simulink model "dq0Invertermeow"  (R2023b)
settings: Solver=VariableStepAuto  StartTime=0.0  StopTime=100  RelTol=1e-3
libraries: eeGeneralControl x7, slpidlib x6, spsAlphaBetaZerotodq0Lib x5, spsCurrentMeasurementLib x5, spsSeriesRLCBranchLib x5, spsIGBTDiodeLib x4, spsabctoAlphaBetaZeroLib x3, spsdq0toAlphaBetaZeroLib x2, spsPLL3phLib x2, simulink x2, spsVoltageMeasurementLib x2, spsACVoltageSourceLib x1
settings Model: Creator=impul  LastModifiedBy=Jia Yee Wong
settings ModelReferenceCC: EnableRefExpFcnMdlSchedulingChecks=on
settings SFSimCC: SimCustomHeaderCode="#include \"referencegen.h\""  SimUserSources=referencegen.c  SimTargetLang=C++

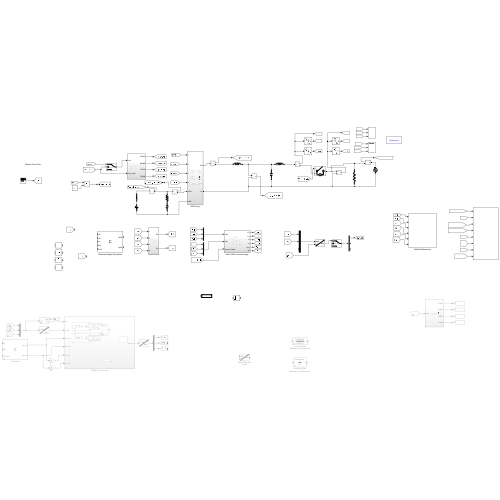
[thumbnail: Simulink's stored preview of the top-level diagram]
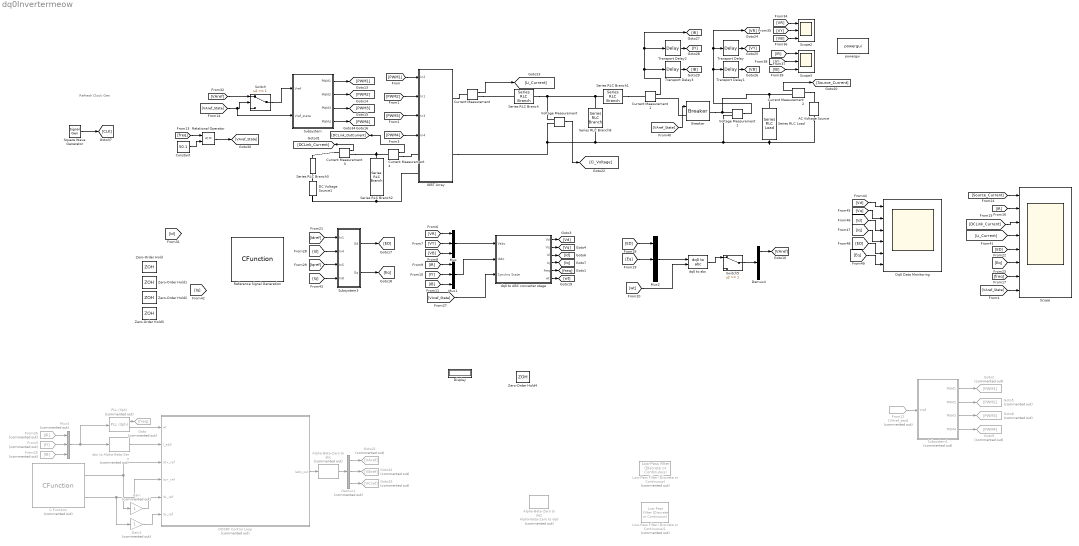
== system dq0Invertermeow ==
  note: Refresh Clock Gen
  AC Voltage Source : spsACVoltageSourceLib/AC Voltage Source  Amplitude=340  Phase=0  Frequency=50  SampleTime=0  Measurements=None  BusType=swing  Pref=0  Qref=0  Qmin=-inf  Qmax=+inf
  Alpha-Beta-Zero to abc : spsAlphaBetaZerotoabcLib/Alpha-Beta-Zero to abc  Commented=on
      settings: LibrarySourceBlock=|
      | sps_lib/Control/Alpha-Beta-Zero
      | to abc
  Alpha-Beta-Zero to dq2 : spsAlphaBetaZerotodq0Lib/Alpha-Beta-Zero to dq0  Commented=on  Alignment=90 degrees behind phase A axis
  Breaker : spsBreakerLib/Breaker  InitialState=0  SwitchingTimes="[1/60  5/60]"  External=on  BreakerResistance=0.00001  SnubberResistance=1e6  SnubberCapacitance=inf  Measurements=None  MoreParameters=on  NoBreakLoop=off
  C Function : CFunction  Commented=on
  Constant : Constant  Value=50.1  SampleTime=0
  Current Measurement{,1..4} (5 alike) : spsCurrentMeasurementLib/Current Measurement  PhasorSimulation=off  OutputType=Complex  PSBequivalent=0
  DC Voltage Source1 : spsDCVoltageSourceLib/DC Voltage Source  Amplitude=400  Measurements=None
  DDSRF Control Loop : Subsystem  Commented=on
  Demux1 : Demux  Commented=on  Outputs=3
  Demux4 : Demux  Outputs=3
  Display : Display
  Dq0 Data Monitoring : Scope  NumInputPorts=6
  From12 : From  Commented=on  GotoTag=VAref_test
  From25 : From  Commented=on  GotoTag=IB
  From26 : From  Commented=on  GotoTag=IR
  From5 : From  Commented=on  GotoTag=IY
  Gain : Gain  Commented=on
  Gain1 : Gain  Commented=on
  Goto : Goto  Commented=on  GotoTag=freq
  Goto2 : Goto  Commented=on  GotoTag=PWM1
  Goto21 : Goto  Commented=on  GotoTag=VAref
  Goto32 : Goto  Commented=on  GotoTag=VBref
  Goto33 : Goto  Commented=on  GotoTag=VCref
  Goto5 : Goto  Commented=on  GotoTag=PWM2
  Goto8 : Goto  Commented=on  GotoTag=PWM3
  Goto9 : Goto  Commented=on  GotoTag=PWM4
  IGBT Array : Subsystem
  Low-Pass Filter (Discrete or Continuous) : eeGeneralControl/Low-Pass Filter (Discrete or Continuous)  Commented=on  K=1  T=2*pi*1  B=inf  A=-inf  init_option=Inherited from block input  x0=0  Ts=0
  Low-Pass Filter (Discrete or Continuous)1 : eeGeneralControl/Low-Pass Filter (Discrete or Continuous)  Commented=on  K=1  T=1  B=inf  A=-inf  init_option=Inherited from block input  x0=0  Ts=0
  Mux : Mux  Inputs=3
  Mux1 : Mux  Inputs=3
  Mux2 : Mux  Inputs=3
  Mux3 : Mux  Commented=on  Inputs=3
  PLL (3ph) : spsPLL3phLib/PLL (3ph)  Commented=on  Fmin=45  Par_Init=[0, 60]  ParK=[180, 3200, 1]  TcD=1e-4  MaxRateChangeFreq=12  FilterCutOffFreq=25  Ts=0  AGC=on
  Reference Signal Generation : CFunction
  Relational Operator : RelationalOperator  Operator=<=  OutDataTypeStr=boolean  RndMeth=Simplest  InputSameDT=off
  Scope : Scope  NumInputPorts=8
  Scope2 : Scope  NumInputPorts=3
  Scope3 : Scope  NumInputPorts=3
  Series RLC Branch : spsSeriesRLCBranchLib/Series RLC Branch  LConnTagsString=__new0  RConnTagsString=__new0  BranchType=L  Resistance=1  Inductance=20.4e-3  SetiL0=off  InitialCurrent=0  Capacitance=1e-6  Setx0=off  InitialVoltage=0  Measurements=None
  Series RLC Branch1 : spsSeriesRLCBranchLib/Series RLC Branch  LConnTagsString=__new0  RConnTagsString=__new0  BranchType=L  Resistance=1  Inductance=148.336e-6  SetiL0=off  InitialCurrent=0  Capacitance=1e-6  Setx0=off  InitialVoltage=0  Measurements=None
  Series RLC Branch2 : spsSeriesRLCBranchLib/Series RLC Branch  LConnTagsString=__new0  RConnTagsString=__new0  BranchType=RC  Resistance=0.1  Inductance=0  SetiL0=off  InitialCurrent=0  Capacitance=1e-6  Setx0=off  InitialVoltage=0  Measurements=None
  Series RLC Branch3 : spsSeriesRLCBranchLib/Series RLC Branch  LConnTagsString=__new0  RConnTagsString=__new0  BranchType=R  Resistance=50  Inductance=0  SetiL0=off  InitialCurrent=0  Capacitance=1e-6  Setx0=off  InitialVoltage=0  Measurements=None
  Series RLC Branch8 : spsSeriesRLCBranchLib/Series RLC Branch  LConnTagsString=__new0  RConnTagsString=__new0  BranchType=C  Resistance=1  Inductance=100e-6  SetiL0=off  InitialCurrent=0  Capacitance=5.526e-6  Setx0=off  InitialVoltage=0  Measurements=None
  Series RLC Load : spsSeriesRLCLoadLib/Series RLC Load  LConnTagsString=a  RConnTagsString=__new0  NominalVoltage=240  NominalFrequency=50  ActivePower=2e3  InductivePower=0  CapacitivePower=0  Setx0=off  InitialVoltage=240  SetiL0=off  InitialCurrent=10  Measurements=None  LoadType=constant PQ
  Square Wave Generator : SignalGenerator  WaveForm=square  Frequency=10e3
  Subsystem : Subsystem
  Subsystem1 : Subsystem  Commented=on
  Subsystem3 : Subsystem
  Switch : Switch  Threshold=1  SaturateOnIntegerOverflow=off  InputSameDT=off
  Switch5 : Switch  Threshold=1  SaturateOnIntegerOverflow=off  InputSameDT=off
  Transport Delay : TransportDelay  DelayTime=6.67e-3  BufferSize=4096
  Transport Delay1 : TransportDelay  DelayTime=13.34e-3  BufferSize=5120
  Transport Delay2 : TransportDelay  DelayTime=6.67e-3  BufferSize=4096
  Transport Delay3 : TransportDelay  DelayTime=13.34e-3  BufferSize=4096
  Voltage Measurement : spsVoltageMeasurementLib/Voltage Measurement  PhasorSimulation=off  OutputType=Complex  PSBequivalent=0
  Voltage Measurement1 : spsVoltageMeasurementLib/Voltage Measurement  PhasorSimulation=off  OutputType=Complex  PSBequivalent=0
  Zero-Order Hold{,1..3} (4 alike) : ZeroOrderHold  SampleTime=-1
  Zero-Order Hold4 : ZeroOrderHold  SampleTime=10e-3
  abc to Alpha-Beta-Zero : spsabctoAlphaBetaZeroLib/abc to Alpha-Beta-Zero  Commented=on
  dq0 to ABC converter stage : Subsystem
  dq0 to abc : spsdq0toabcLib/dq0 to abc  Alignment=90 degrees behind phase A axis
  powergui : spspowerguiLib/powergui  Priority=1  SimulationMode=Continuous  SampleTime=50e-6  frequency=60  Iterations=50  frequencyindice=0  Pbase=100e6  ErrMax=1e-4  UnitsV=kV  UnitsW=MW  buscounter=0  FunctionMessages=off  echomessages=off  EnableUseOfTLC=off  CurrentSourceSwitches=off  DisableSnubberDevices=off  DisableRonSwitches=off  DisableVfSwitches=off  DisplayEquations=off  AutomaticDiscreteSolvers=off  SolverType=Tustin/Backward Euler (TBE)  Interpol=off  ExternalGateDelay=off  methode=off  Ts=100  x0status=blocks  SPID=on  SwTol=0  HookPort=off  NonlinearTolerance=1e-4  nMaxIteration=100  ContinueOnMaxIteration=off  RestoreLinks=warning  ResistiveCurrentMeasurement=off  Frange=[0:2:500]  Ylog=off  Xlog=on  ShowGrid=off  save=off  variable=ZData  structure=0  ZoomFFT=off  StartTime=0.0  cycles=1  DisplayStyle=1  fundamental=60  FreqAxis=off  MaxFrequency=1000  frequencyindicesteady=1  RmsSteady=1  display=off
  wires:
  [PWM1] -> IGBT Array/1(In2)
  [PWM2] -> IGBT Array/2(In1)
  [PWM3] -> IGBT Array/3(In3)
  [PWM4] -> IGBT Array/4(In4)
  [ED] -> Mux2/1
  [Eq] -> Mux2/2
  [wt] -> dq0 to abc/2
  Mux2/1 -> dq0 to abc/1
  Demux4/1 -> [VAref]
  Voltage Measurement/1 -> [Ci_Voltage]
  Transport Delay1/1 -> [VB]
  Transport Delay/1 -> [VY]
  Subsystem/1(PWM1) -> [PWM1]
  Subsystem/2(PWM2) -> [PWM2]
  Subsystem/3(PWM3) -> [PWM3]
  Subsystem/4(PWM4) -> [PWM4]
  Transport Delay2/1 -> [IY]
  Transport Delay3/1 -> [IB]
  Current Measurement/1 -> [Li_Current]
  Current Measurement1/1 -> [IR], Transport Delay2/1, Transport Delay3/1
  Current Measurement2/1 -> [Source_Current]
  Subsystem1/2(PWM2) -> Goto5/1
  From12/1 -> Subsystem1/1(Vref)
  Subsystem1/4(PWM4) -> Goto9/1
  Subsystem1/3(PWM3) -> Goto8/1
  Subsystem1/1(PWM1) -> Goto2/1
  Voltage Measurement1/1 -> [VR], Transport Delay/1, Transport Delay1/1
  [VAref] -> Switch/1
  [freq] -> Relational Operator/1
  Constant/1 -> Relational Operator/2
  Current Measurement3/1 -> [DCLink_Current]
  [Eq] -> Scope/6
  [ED] -> Scope/5
  [VAref_State] -> Scope/8
  Switch/1 -> Subsystem/1(Vref)
  [VAref_State] -> Subsystem/2(Vref_state), Switch/2
  [Source_Current] -> Scope/1
  Switch5/1 -> Demux4/1
  dq0 to abc/1 -> Switch5/1
  [VR] -> Scope2/1
  [VY] -> Scope2/2
  [VB] -> Scope2/3
  [IR] -> Scope3/1
  [IY] -> Scope3/2
  [IB] -> Scope3/3
  [Vd] -> Dq0 Data Monitoring/1
  [Vq] -> Dq0 Data Monitoring/2
  [Id] -> Dq0 Data Monitoring/3
  [Iq] -> Dq0 Data Monitoring/4
  [ED] -> Dq0 Data Monitoring/5
  [Eq] -> Dq0 Data Monitoring/6
  [VAref_State] -> Breaker/1
  [freq] -> Scope/7
  [Li_Current] -> Scope/4
  [IR] -> Scope/2
  [DCLink_Current] -> Scope/3
  Relational Operator/1 -> [VAref_State]
  Subsystem3/1(Ed) -> [ED]
  Subsystem3/2(Eq) -> [Eq]
  [VR] -> Mux/1
  [VB] -> Mux/3
  [IB] -> Mux1/3
  Mux1/1 -> dq0 to ABC converter stage/2(IAbc)
  [IY] -> Mux1/2
  Mux/1 -> dq0 to ABC converter stage/1(Vabc)
  [IR] -> Mux1/1
  [VY] -> Mux/2
  dq0 to ABC converter stage/2(Vq) -> [Vq]
  dq0 to ABC converter stage/1(Vd) -> [Vd]
  dq0 to ABC converter stage/3(Id) -> [Id]
  dq0 to ABC converter stage/4(Iq) -> [Iq]
  dq0 to ABC converter stage/6(wt) -> [wt]
  dq0 to ABC converter stage/5(freq) -> [freq]
  DDSRF Control Loop/1(Iabc_out) -> Alpha-Beta-Zero to abc/1
  PLL (3ph)/2 -> DDSRF Control Loop/1(wt)
  PLL (3ph)/1 -> Goto/1
  abc to Alpha-Beta-Zero/1 -> DDSRF Control Loop/2(I_ab0)
  From25/1 -> Mux3/3
  Mux3/1 -> PLL (3ph)/1, abc to Alpha-Beta-Zero/1
  From5/1 -> Mux3/2
  From26/1 -> Mux3/1
  C Function/2 -> Gain1/1, DDSRF Control Loop/4(Iq+_ref)
  Gain/1 -> DDSRF Control Loop/5(Id-_ref)
  C Function/1 -> Gain/1, DDSRF Control Loop/3(Id+_ref)
  Gain1/1 -> DDSRF Control Loop/6(Iq-_ref)
  Demux1/3 -> Goto33/1
  Demux1/2 -> Goto32/1
  Demux1/1 -> Goto21/1
  Alpha-Beta-Zero to abc/1 -> Demux1/1
  [VAref_State] -> dq0 to ABC converter stage/3(Synchro State)
  Current Measurement4/1 -> [DCLink_OutCurrent]
  [Idref] -> Subsystem3/1(In1)
  [Id] -> Subsystem3/2(In4)
  [Iqref] -> Subsystem3/3(In5)
  [Iq] -> Subsystem3/4(In8)
  Square Wave Generator/1 -> [CLK]
  connections:
  Series RLC Branch/RConn1 -- Voltage Measurement/LConn1 -- Series RLC Branch8/LConn1 -- Series RLC Branch1/LConn1
  Series RLC Branch2/RConn1 -- DC Voltage Source1/LConn1 -- IGBT Array/LConn2
  IGBT Array/RConn2 -- Voltage Measurement/LConn2 -- AC Voltage Source/LConn1 -- Series RLC Load/RConn1 -- Voltage Measurement1/LConn2 -- Series RLC Branch8/RConn1
  IGBT Array/RConn1 -- Current Measurement/LConn1
  Current Measurement/RConn1 -- Series RLC Branch/LConn1
  Series RLC Branch1/RConn1 -- Current Measurement1/LConn1
  Current Measurement2/LConn1 -- AC Voltage Source/RConn1
  Current Measurement2/RConn1 -- Breaker/RConn1 -- Voltage Measurement1/LConn1 -- Series RLC Load/LConn1
  Current Measurement3/RConn1 -- Series RLC Branch2/LConn1 -- Current Measurement4/LConn1
  Series RLC Branch3/RConn1 -- DC Voltage Source1/RConn1
  Breaker/LConn1 -- Current Measurement1/RConn1
  Current Measurement3/LConn1 -- Series RLC Branch3/LConn1
  Current Measurement4/RConn1 -- IGBT Array/LConn1

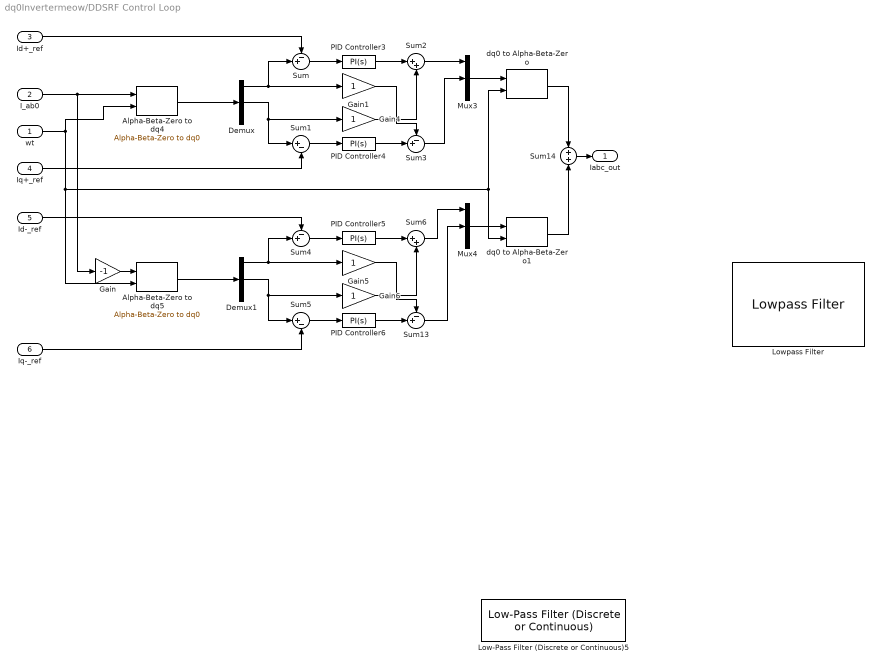
== system dq0Invertermeow/DDSRF Control Loop ==
  wt : Inport
  I_ab0 : Inport  Port=2
  Id+_ref : Inport  Port=3
  Iq+_ref : Inport  Port=4
  Id-_ref : Inport  Port=5
  Iq-_ref : Inport  Port=6
  Alpha-Beta-Zero to dq4 : spsAlphaBetaZerotodq0Lib/Alpha-Beta-Zero to dq0  Alignment=90 degrees behind phase A axis
  Alpha-Beta-Zero to dq5 : spsAlphaBetaZerotodq0Lib/Alpha-Beta-Zero to dq0  Alignment=90 degrees behind phase A axis
  Demux : Demux  Outputs=3
  Demux1 : Demux  Outputs=3
  Gain : Gain  Gain=-1
  Gain{1,4..6} (4 alike) : Gain
  Low-Pass Filter (Discrete or Continuous)5 : eeGeneralControl/Low-Pass Filter (Discrete or Continuous)  K=1  T=2*pi*50  B=inf  A=-inf  init_option=Inherited from block input  x0=0  Ts=0
  Lowpass Filter : dspfdesign/Lowpass Filter  FilterType=FIR  DesignForMinimumOrder=on  FilterOrder=50  PassbandFrequency=8e3  StopbandFrequency=12e3  PassbandRipple=0.1  StopbandAttenuation=80  SampleRateMode=Specify on dialog  SampleRate=44100  SimulateUsing=Interpreted execution  roundingMode=Floor  coeffsDataTypeStr=fixdt(1,16)
  Mux3 : Mux  Inputs=3
  Mux4 : Mux  Inputs=3
  PID Controller{3..6} (4 alike) : slpidlib/PID Controller  Controller=PI  Form=Parallel  TimeDomain=Continuous-time  UseExternalTs=off  SampleTime=-1  IntegratorMethod=Forward Euler  FilterMethod=Forward Euler  ControllerParametersSource=internal  P=1  I=1  UseKiTs=off  D=0  N=100  UseFilter=on  TunerSelectOption=Transfer Function Based (PID Tuner App)  InitialConditionSource=internal  InitialConditionForIntegrator=0  InitialConditionForFilter=0  DifferentiatorICPrevScaledInput=0  ExternalReset=none  TrackingMode=off  Kt=1  LimitOutput=off  SatLimitsSource=internal  UpperSaturationLimit=inf  LowerSaturationLimit=-inf  LinearizeAsGain=on  AntiWindupMode=none  Kb=1  LimitIntegrator=off  UpperIntegratorSaturationLimit=inf  LowerIntegratorSaturationLimit=-inf  POutMin=[]  POutMax=[]  IOutMin=[]  IOutMax=[]  DOutMin=[]  DOutMax=[]  NOutMin=[]  NOutMax=[]  SumOutMin=[]  SumOutMax=[]  SaturationOutMin=[]  SaturationOutMax=[]  PParamMin=[]  PParamMax=[]  IParamMin=[]  IParamMax=[]  DParamMin=[]  DParamMax=[]  NParamMin=[]  NParamMax=[]  KbParamMin=[]  KbParamMax=[]  KtParamMin=[]  KtParamMax=[]  KbOutMin=[]  KbOutMax=[]  KtOutMin=[]  KtOutMax=[]  IntegratorOutMin=[]  IntegratorOutMax=[]  FilterOutMin=[]  FilterOutMax=[]  SumI1OutMin=[]  SumI1OutMax=[]  SumI2OutMin=[]  SumI2OutMax=[]  SumI3OutMin=[]  SumI3OutMax=[]  SumI4OutMin=[]  SumI4OutMax=[]  SumDOutMin=[]  SumDOutMax=[]  DifferentiatorOutMin=[]  DifferentiatorOutMax=[]  FilterDiffOutCoefMin=[]  FilterDiffOutCoefMax=[]  ReciprocalOutMin=[]  ReciprocalOutMax=[]  SumDenOutMin=[]  SumDenOutMax=[]  SumNumOutMin=[]  SumNumOutMax=[]  DivideOutMin=[]  DivideOutMax=[]  UdiffTsProdOutMin=[]  UdiffTsProdOutMax=[]  NTsProdOutMin=[]  NTsProdOutMax=[]  UintegralTsProdOutMin=[]  UintegralTsProdOutMax=[]  UngainTsProdOutMin=[]  UngainTsProdOutMax=[]  ClampingZeroOutDataTypeStr=Inherit: Inherit via back propagation  ClampingZeroOutMin=[]  ClampingZeroOutMax=[]  FilterDenConstantOutDataTypeStr=Inherit: Inherit via back propagation  FilterDenConstantOutMin=[]  FilterDenConstantOutMax=[]  PCopyOutDataTypeStr=Inherit: Inherit via back propagation  PCopyOutMin=[]  PCopyOutMax=[]  NCopyOutDataTypeStr=Inherit: Inherit via back propagation  NCopyOutMin=[]  NCopyOutMax=[]  IntegratorContinuousStateAttributes=''  IntegratorStateMustResolveToSignalObject=off  IntegratorRTWStateStorageClass=Auto  FilterContinuousStateAttributes=''  FilterStateMustResolveToSignalObject=off  FilterRTWStateStorageClass=Auto  ParallelPVariant=InternalParameters  IdealPVariant=Disabled  IVariant=InternalParameters  DVariant=Disabled  IntegratorVariant=Continuous  SatVariant=Disabled  AWVariant=Passthrough  PCopyVariant=Disabled  TRVariant=Disabled  FdbkBlocksVariant=Forward  IdealPFdbkVariant=Disabled  SatFdbkVariant=Disabled  DerivativeFilterVariant=Disabled  NVariant=Disabled  NCopyVariant=Disabled_SignalSpec  FilterICVariant=Disabled  IntegratorICVariant=InternalICs  ExternalResetVariant=Disabled  TRSumVariant=Passthrough  SumFdbkVariant=Disabled  SumVariant=Sum_PI  TsampFilterVariant=InternalTs  TsampNgainVariant=Passthrough  TsampIntegralVariant=Disabled_SignalSpec  ExternalSaturationOutDataTypeStr=Inherit: Same as second input
  Sum{,3..4,13} (4 alike) : Sum  Inputs=-+|
  Sum1 : Sum  Inputs=|+-
  Sum14 : Sum  Inputs=+|+
  Sum2 : Sum  Inputs=|++
  Sum5 : Sum  Inputs=|+-
  Sum6 : Sum  Inputs=|++
  dq0 to Alpha-Beta-Zero : spsdq0toAlphaBetaZeroLib/dq0 to Alpha-Beta-Zero  Alignment=90 degrees behind phase A axis
  dq0 to Alpha-Beta-Zero1 : spsdq0toAlphaBetaZeroLib/dq0 to Alpha-Beta-Zero  Alignment=90 degrees behind phase A axis
  Iabc_out : Outport
  wires:
  Gain/1 -> Alpha-Beta-Zero to dq5/1
  Gain5/1 -> Sum13/1
  Mux3/1 -> dq0 to Alpha-Beta-Zero/1
  PID Controller3/1 -> Sum2/1
  Id-_ref/1 -> Sum4/1
  Demux1/1 -> Gain5/1, Sum4/2
  Demux/1 -> Gain1/1, Sum/2
  Demux/2 -> Gain4/1, Sum1/1
  Sum4/1 -> PID Controller5/1
  dq0 to Alpha-Beta-Zero/1 -> Sum14/1
  PID Controller6/1 -> Sum13/2
  Demux1/2 -> Gain6/1, Sum5/1
  Alpha-Beta-Zero to dq4/1 -> Demux/1
  PID Controller4/1 -> Sum3/2
  Mux4/1 -> dq0 to Alpha-Beta-Zero1/1
  Id+_ref/1 -> Sum/1
  Gain1/1 -> Sum3/1
  Sum/1 -> PID Controller3/1
  Sum1/1 -> PID Controller4/1
  Sum6/1 -> Mux4/1
  Sum2/1 -> Mux3/1
  Iq-_ref/1 -> Sum5/2
  I_ab0/1 -> Alpha-Beta-Zero to dq4/1, Gain/1
  Iq+_ref/1 -> Sum1/2
  Sum3/1 -> Mux3/2
  wt/1 -> Alpha-Beta-Zero to dq4/2, dq0 to Alpha-Beta-Zero/2, dq0 to Alpha-Beta-Zero1/2, Alpha-Beta-Zero to dq5/2
  Alpha-Beta-Zero to dq5/1 -> Demux1/1
  Sum5/1 -> PID Controller6/1
  dq0 to Alpha-Beta-Zero1/1 -> Sum14/2
  Gain6/1 -> Sum6/2
  Sum13/1 -> Mux4/2
  Gain4/1 -> Sum2/2
  PID Controller5/1 -> Sum6/1
  Sum14/1 -> Iabc_out/1

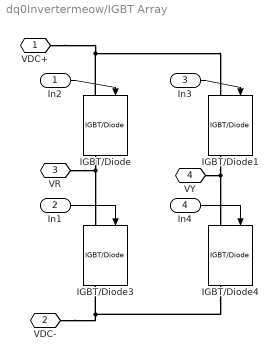
== system dq0Invertermeow/IGBT Array ==
  In2 : Inport
  In1 : Inport  Port=2
  In3 : Inport  Port=3
  In4 : Inport  Port=4
  IGBT/Diode{,1,3..4} (4 alike) : spsIGBTDiodeLib/IGBT//Diode  Ron=1e-3  Rs=1e5  Cs=inf  Measurements=on
  VDC+ : PMIOPort  Side=Left
  VDC- : PMIOPort  Port=2  Side=Left
  VR : PMIOPort  Port=3  Side=Right
  VY : PMIOPort  Port=4  Side=Right
  wires:
  In1/1 -> IGBT/Diode3/1
  In4/1 -> IGBT/Diode4/1
  In3/1 -> IGBT/Diode1/1
  In2/1 -> IGBT/Diode/1
  connections:
  IGBT/Diode4/RConn1 -- VDC-/RConn1 -- IGBT/Diode3/RConn1
  IGBT/Diode/RConn1 -- VR/RConn1 -- IGBT/Diode3/LConn1
  IGBT/Diode1/RConn1 -- VY/RConn1 -- IGBT/Diode4/LConn1
  IGBT/Diode/LConn1 -- VDC+/RConn1 -- IGBT/Diode1/LConn1

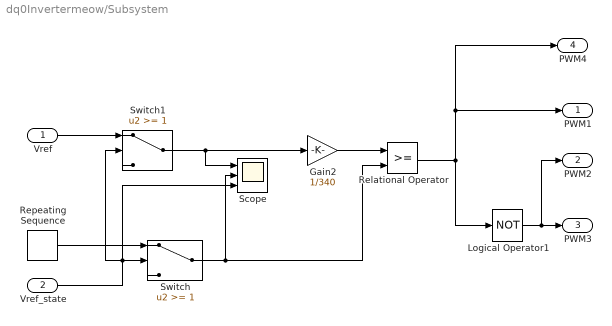
== system dq0Invertermeow/Subsystem ==
  Vref : Inport
  Vref_state : Inport  Port=2
  Gain2 : Gain  Gain=1/340
  Logical Operator1 : Logic  Operator=NOT  AllPortsSameDT=off  OutDataTypeStr=boolean
  Relational Operator : RelationalOperator  OutDataTypeStr=boolean  RndMeth=Simplest  InputSameDT=off
  Repeating Sequence : simulink/Sources/Repeating Sequence  rep_seq_t=[0 0.00005 0.0001]  rep_seq_y=[-1 1 -1]
  Scope : Scope  NumInputPorts=3
  Switch : Switch  Threshold=1  SaturateOnIntegerOverflow=off  InputSameDT=off
  Switch1 : Switch  Threshold=1  SaturateOnIntegerOverflow=off  InputSameDT=off
  PWM1 : Outport
  PWM2 : Outport  Port=2
  PWM3 : Outport  Port=3
  PWM4 : Outport  Port=4
  wires:
  Gain2/1 -> Relational Operator/1
  Relational Operator/1 -> Logical Operator1/1, PWM1/1, PWM4/1
  Logical Operator1/1 -> PWM2/1, PWM3/1
  Repeating Sequence/1 -> Switch/1
  Switch/1 -> Scope/2, Relational Operator/2
  Vref_state/1 -> Scope/3, Switch1/2, Switch/2
  Switch1/1 -> Gain2/1, Scope/1
  Vref/1 -> Switch1/1

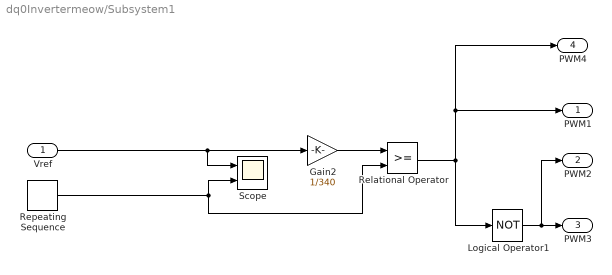
== system dq0Invertermeow/Subsystem1 ==
  Vref : Inport
  Gain2 : Gain  Gain=1/340
  Logical Operator1 : Logic  Operator=NOT  AllPortsSameDT=off  OutDataTypeStr=boolean
  Relational Operator : RelationalOperator  OutDataTypeStr=boolean  RndMeth=Simplest  InputSameDT=off
  Repeating Sequence : simulink/Sources/Repeating Sequence  rep_seq_t=[0 0.00005 0.0001]  rep_seq_y=[-1 1 -1]
  Scope : Scope  NumInputPorts=2
  PWM1 : Outport
  PWM2 : Outport  Port=2
  PWM3 : Outport  Port=3
  PWM4 : Outport  Port=4
  wires:
  Repeating Sequence/1 -> Scope/2, Relational Operator/2
  Gain2/1 -> Relational Operator/1
  Relational Operator/1 -> Logical Operator1/1, PWM1/1, PWM4/1
  Logical Operator1/1 -> PWM2/1, PWM3/1
  Vref/1 -> Scope/1, Gain2/1

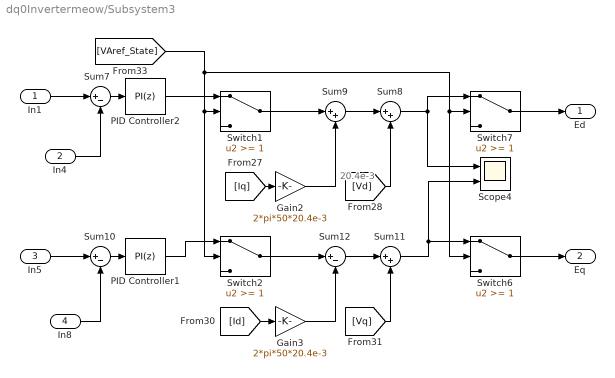
== system dq0Invertermeow/Subsystem3 ==
  note: 20.4e-3
  In1 : Inport
  In4 : Inport  Port=2
  In5 : Inport  Port=3
  In8 : Inport  Port=4
  Gain2 : Gain  Gain=2*pi*50*20.4e-3
  Gain3 : Gain  Gain=2*pi*50*20.4e-3
  PID Controller1 : slpidlib/PID Controller  Controller=PI  Form=Ideal  TimeDomain=Discrete-time  UseExternalTs=off  SampleTime=1e-4  IntegratorMethod=Forward Euler  FilterMethod=Forward Euler  ControllerParametersSource=internal  P=10  I=0.07  UseKiTs=on  D=0.2  N=100  UseFilter=on  TunerSelectOption=Transfer Function Based (PID Tuner App)  InitialConditionSource=internal  InitialConditionForIntegrator=0  InitialConditionForFilter=0  DifferentiatorICPrevScaledInput=0  ExternalReset=none  TrackingMode=off  Kt=1  LimitOutput=on  SatLimitsSource=internal  UpperSaturationLimit=200  LowerSaturationLimit=-200  LinearizeAsGain=on  AntiWindupMode=clamping  Kb=1  LimitIntegrator=off  UpperIntegratorSaturationLimit=inf  LowerIntegratorSaturationLimit=-inf  POutMin=[]  POutMax=[]  IOutMin=[]  IOutMax=[]  DOutMin=[]  DOutMax=[]  NOutMin=[]  NOutMax=[]  SumOutMin=[]  SumOutMax=[]  SaturationOutMin=[]  SaturationOutMax=[]  PParamMin=[]  PParamMax=[]  IParamMin=[]  IParamMax=[]  DParamMin=[]  DParamMax=[]  NParamMin=[]  NParamMax=[]  KbParamMin=[]  KbParamMax=[]  KtParamMin=[]  KtParamMax=[]  KbOutMin=[]  KbOutMax=[]  KtOutMin=[]  KtOutMax=[]  IntegratorOutMin=[]  IntegratorOutMax=[]  FilterOutMin=[]  FilterOutMax=[]  SumI1OutMin=[]  SumI1OutMax=[]  SumI2OutMin=[]  SumI2OutMax=[]  SumI3OutMin=[]  SumI3OutMax=[]  SumI4OutMin=[]  SumI4OutMax=[]  SumDOutMin=[]  SumDOutMax=[]  DifferentiatorOutMin=[]  DifferentiatorOutMax=[]  FilterDiffOutCoefMin=[]  FilterDiffOutCoefMax=[]  ReciprocalOutMin=[]  ReciprocalOutMax=[]  SumDenOutMin=[]  SumDenOutMax=[]  SumNumOutMin=[]  SumNumOutMax=[]  DivideOutMin=[]  DivideOutMax=[]  UdiffTsProdOutMin=[]  UdiffTsProdOutMax=[]  NTsProdOutMin=[]  NTsProdOutMax=[]  UintegralTsProdOutMin=[]  UintegralTsProdOutMax=[]  UngainTsProdOutMin=[]  UngainTsProdOutMax=[]  ClampingZeroOutDataTypeStr=Inherit: Inherit via back propagation  ClampingZeroOutMin=[]  ClampingZeroOutMax=[]  FilterDenConstantOutDataTypeStr=Inherit: Inherit via back propagation  FilterDenConstantOutMin=[]  FilterDenConstantOutMax=[]  PCopyOutDataTypeStr=Inherit: Inherit via back propagation  PCopyOutMin=[]  PCopyOutMax=[]  NCopyOutDataTypeStr=Inherit: Inherit via back propagation  NCopyOutMin=[]  NCopyOutMax=[]  IntegratorContinuousStateAttributes=''  IntegratorStateMustResolveToSignalObject=off  IntegratorRTWStateStorageClass=Auto  FilterContinuousStateAttributes=''  FilterStateMustResolveToSignalObject=off  FilterRTWStateStorageClass=Auto  ParallelPVariant=Passthrough  IdealPVariant=InternalParameters  IVariant=InternalParameters  DVariant=Disabled  IntegratorVariant=Discrete  SatVariant=Enabled  AWVariant=DiscClampingIdeal  PCopyVariant=InternalParamsIdeal  TRVariant=Disabled  FdbkBlocksVariant=Forward  IdealPFdbkVariant=Disabled  SatFdbkVariant=Disabled  DerivativeFilterVariant=Disabled  NVariant=Disabled  NCopyVariant=Disabled_SignalSpec  FilterICVariant=Disabled  IntegratorICVariant=InternalICs  ExternalResetVariant=Disabled  TRSumVariant=Passthrough  SumFdbkVariant=Disabled  SumVariant=Sum_PI  TsampFilterVariant=InternalTs  TsampNgainVariant=Passthrough  TsampIntegralVariant=Disabled_SignalSpec  ExternalSaturationOutDataTypeStr=Inherit: Same as second input
  PID Controller2 : slpidlib/PID Controller  Controller=PI  Form=Parallel  TimeDomain=Discrete-time  UseExternalTs=off  SampleTime=1e-4  IntegratorMethod=Forward Euler  FilterMethod=Forward Euler  ControllerParametersSource=internal  P=10  I=0.07  UseKiTs=on  D=0.2  N=100  UseFilter=on  TunerSelectOption=Transfer Function Based (PID Tuner App)  InitialConditionSource=internal  InitialConditionForIntegrator=0  InitialConditionForFilter=0  DifferentiatorICPrevScaledInput=0  ExternalReset=none  TrackingMode=off  Kt=1  LimitOutput=on  SatLimitsSource=internal  UpperSaturationLimit=200  LowerSaturationLimit=-200  LinearizeAsGain=on  AntiWindupMode=back-calculation  Kb=1  LimitIntegrator=off  UpperIntegratorSaturationLimit=inf  LowerIntegratorSaturationLimit=-inf  POutMin=[]  POutMax=[]  IOutMin=[]  IOutMax=[]  DOutMin=[]  DOutMax=[]  NOutMin=[]  NOutMax=[]  SumOutMin=[]  SumOutMax=[]  SaturationOutMin=[]  SaturationOutMax=[]  PParamMin=[]  PParamMax=[]  IParamMin=[]  IParamMax=[]  DParamMin=[]  DParamMax=[]  NParamMin=[]  NParamMax=[]  KbParamMin=[]  KbParamMax=[]  KtParamMin=[]  KtParamMax=[]  KbOutMin=[]  KbOutMax=[]  KtOutMin=[]  KtOutMax=[]  IntegratorOutMin=[]  IntegratorOutMax=[]  FilterOutMin=[]  FilterOutMax=[]  SumI1OutMin=[]  SumI1OutMax=[]  SumI2OutMin=[]  SumI2OutMax=[]  SumI3OutMin=[]  SumI3OutMax=[]  SumI4OutMin=[]  SumI4OutMax=[]  SumDOutMin=[]  SumDOutMax=[]  DifferentiatorOutMin=[]  DifferentiatorOutMax=[]  FilterDiffOutCoefMin=[]  FilterDiffOutCoefMax=[]  ReciprocalOutMin=[]  ReciprocalOutMax=[]  SumDenOutMin=[]  SumDenOutMax=[]  SumNumOutMin=[]  SumNumOutMax=[]  DivideOutMin=[]  DivideOutMax=[]  UdiffTsProdOutMin=[]  UdiffTsProdOutMax=[]  NTsProdOutMin=[]  NTsProdOutMax=[]  UintegralTsProdOutMin=[]  UintegralTsProdOutMax=[]  UngainTsProdOutMin=[]  UngainTsProdOutMax=[]  ClampingZeroOutDataTypeStr=Inherit: Inherit via back propagation  ClampingZeroOutMin=[]  ClampingZeroOutMax=[]  FilterDenConstantOutDataTypeStr=Inherit: Inherit via back propagation  FilterDenConstantOutMin=[]  FilterDenConstantOutMax=[]  PCopyOutDataTypeStr=Inherit: Inherit via back propagation  PCopyOutMin=[]  PCopyOutMax=[]  NCopyOutDataTypeStr=Inherit: Inherit via back propagation  NCopyOutMin=[]  NCopyOutMax=[]  IntegratorContinuousStateAttributes=''  IntegratorStateIdentifier=Id  IntegratorStateMustResolveToSignalObject=off  IntegratorRTWStateStorageClass=Auto  FilterContinuousStateAttributes=''  FilterStateMustResolveToSignalObject=off  FilterRTWStateStorageClass=Auto  ParallelPVariant=InternalParameters  IdealPVariant=Disabled  IVariant=InternalParameters  DVariant=Disabled  IntegratorVariant=Discrete  SatVariant=Enabled  AWVariant=BackCalculation  PCopyVariant=Disabled  TRVariant=Disabled  FdbkBlocksVariant=Forward  IdealPFdbkVariant=Disabled  SatFdbkVariant=Disabled  DerivativeFilterVariant=Disabled  NVariant=Disabled  NCopyVariant=Disabled_SignalSpec  FilterICVariant=Disabled  IntegratorICVariant=InternalICs  ExternalResetVariant=Disabled  TRSumVariant=Passthrough  SumFdbkVariant=Disabled  SumVariant=Sum_PI  TsampFilterVariant=InternalTs  TsampNgainVariant=Passthrough  TsampIntegralVariant=Disabled_SignalSpec  ExternalSaturationOutDataTypeStr=Inherit: Same as second input
  Scope4 : Scope  NumInputPorts=2
  Sum10 : Sum  Inputs=|+-
  Sum11 : Sum  Inputs=|++
  Sum12 : Sum  Inputs=|+-
  Sum7 : Sum  Inputs=|+-
  Sum8 : Sum  Inputs=|++
  Sum9 : Sum  Inputs=|++
  Switch{1..2,6..7} (4 alike) : Switch  Threshold=1  SaturateOnIntegerOverflow=off  InputSameDT=off
  Ed : Outport
  Eq : Outport  Port=2
  wires:
  Switch1/1 -> Sum9/1
  In5/1 -> Sum10/1
  In1/1 -> Sum7/1
  [Vq] -> Sum11/2
  [VAref_State] -> Switch6/2, Switch7/2, Switch2/2, Switch1/2
  Switch7/1 -> Ed/1
  In4/1 -> Sum7/2
  Sum8/1 -> Scope4/1, Switch7/1
  Sum10/1 -> PID Controller1/1
  Sum11/1 -> Switch6/1, Scope4/2
  In8/1 -> Sum10/2
  Gain3/1 -> Sum12/2
  Sum7/1 -> PID Controller2/1
  PID Controller1/1 -> Switch2/1
  [Vd] -> Sum8/2
  Sum9/1 -> Sum8/1
  Gain2/1 -> Sum9/2
  Sum12/1 -> Sum11/1
  [Iq] -> Gain2/1
  [Id] -> Gain3/1
  PID Controller2/1 -> Switch1/1
  Switch2/1 -> Sum12/1
  Switch6/1 -> Eq/1

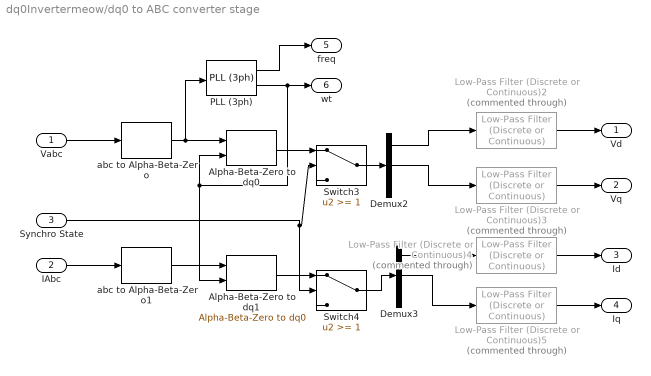
== system dq0Invertermeow/dq0 to ABC converter stage ==
  Vabc : Inport
  IAbc : Inport  Port=2
  Synchro State : Inport  Port=3
  Alpha-Beta-Zero to dq0 : spsAlphaBetaZerotodq0Lib/Alpha-Beta-Zero to dq0  Alignment=90 degrees behind phase A axis
  Alpha-Beta-Zero to dq1 : spsAlphaBetaZerotodq0Lib/Alpha-Beta-Zero to dq0  Alignment=90 degrees behind phase A axis
  Demux2 : Demux  Outputs=3
  Demux3 : Demux  Outputs=3
  Low-Pass Filter (Discrete or Continuous){2..5} (4 alike) : eeGeneralControl/Low-Pass Filter (Discrete or Continuous)  Commented=through  K=1  T=2*pi*50  B=inf  A=-inf  init_option=Inherited from block input  x0=0  Ts=0
  PLL (3ph) : spsPLL3phLib/PLL (3ph)  Fmin=45  Par_Init=[0, 60]  ParK=[180, 3200, 1]  TcD=1e-4  MaxRateChangeFreq=12  FilterCutOffFreq=25  Ts=0  AGC=on
  Switch3 : Switch  Threshold=1  SaturateOnIntegerOverflow=off  InputSameDT=off
  Switch4 : Switch  Threshold=1  SaturateOnIntegerOverflow=off  InputSameDT=off
  abc to Alpha-Beta-Zero : spsabctoAlphaBetaZeroLib/abc to Alpha-Beta-Zero
  abc to Alpha-Beta-Zero1 : spsabctoAlphaBetaZeroLib/abc to Alpha-Beta-Zero
  Vd : Outport
  Vq : Outport  Port=2
  Id : Outport  Port=3
  Iq : Outport  Port=4
  freq : Outport  Port=5
  wt : Outport  Port=6
  wires:
  Demux3/2 -> Low-Pass Filter (Discrete or Continuous)5/1
  Synchro State/1 -> Switch4/2, Switch3/2
  Demux3/1 -> Low-Pass Filter (Discrete or Continuous)4/1
  Low-Pass Filter (Discrete or Continuous)5/1 -> Iq/1
  abc to Alpha-Beta-Zero1/1 -> Alpha-Beta-Zero to dq1/1
  Low-Pass Filter (Discrete or Continuous)4/1 -> Id/1
  Switch4/1 -> Demux3/1
  Demux2/2 -> Low-Pass Filter (Discrete or Continuous)3/1
  Low-Pass Filter (Discrete or Continuous)2/1 -> Vd/1
  Alpha-Beta-Zero to dq1/1 -> Switch4/1
  Demux2/1 -> Low-Pass Filter (Discrete or Continuous)2/1
  Low-Pass Filter (Discrete or Continuous)3/1 -> Vq/1
  Switch3/1 -> Demux2/1
  PLL (3ph)/1 -> freq/1
  Alpha-Beta-Zero to dq0/1 -> Switch3/1
  abc to Alpha-Beta-Zero/1 -> PLL (3ph)/1, Alpha-Beta-Zero to dq0/1
  Vabc/1 -> abc to Alpha-Beta-Zero/1
  PLL (3ph)/2 -> Alpha-Beta-Zero to dq1/2, Alpha-Beta-Zero to dq0/2, wt/1
  IAbc/1 -> abc to Alpha-Beta-Zero1/1
